simulink model "pid_model"  (R2020b)
settings: Solver=VariableStepAuto  StartTime=0.0  StopTime=5.0  RelTol=1e-3
undefined symbols (not defined in the file or in its folder): control, k_d, k_i, k_p, k_v, position_output, position_setpoint, sample_time, tau_s
settings Model: Creator=wmmc88  LastModifiedBy=wmmc88

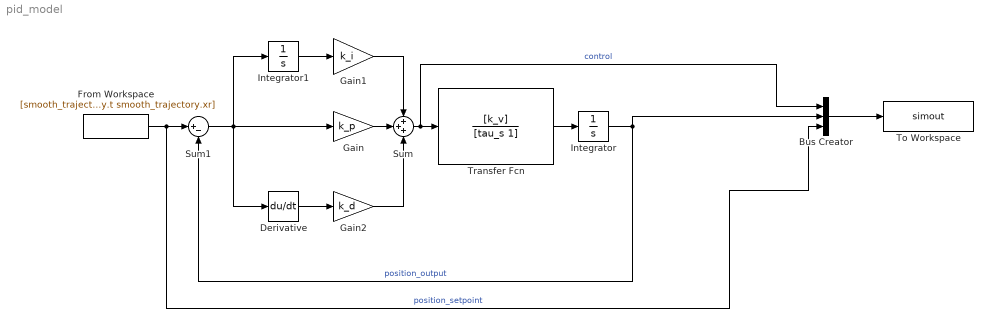
== system pid_model ==
  Bus Creator : BusCreator  Inputs=control,position_output,position_setpoint
  Derivative : Derivative
  From Workspace : FromWorkspace  VariableName=[smooth_trajectory.t smooth_trajectory.xr]  SampleTime=sample_time  ZeroCross=off  OutputAfterFinalValue=Setting to zero
  Gain : Gain  Gain=k_p
  Gain1 : Gain  Gain=k_i
  Gain2 : Gain  Gain=k_d
  Integrator : Integrator
  Integrator1 : Integrator
  Sum : Sum  Inputs=+++
  Sum1 : Sum  Inputs=|+-
  To Workspace : ToWorkspace  VariableName=simout  SaveFormat=Timeseries  SampleTime=sample_time
  Transfer Fcn : TransferFcn  Numerator=[k_v]  Denominator=[tau_s 1]
  wires:
  Bus Creator/1 -> To Workspace/1
  Transfer Fcn/1 -> Integrator/1
  Sum/1 -> Bus Creator/1, Transfer Fcn/1  "control"
  Gain2/1 -> Sum/3
  Gain/1 -> Sum/2
  Gain1/1 -> Sum/1
  Sum1/1 -> Derivative/1, Integrator1/1, Gain/1
  Integrator/1 -> Bus Creator/2, Sum1/2  "position_output"
  Integrator1/1 -> Gain1/1
  Derivative/1 -> Gain2/1
  From Workspace/1 -> Bus Creator/3, Sum1/1  "position_setpoint"
